simulink model "finaltuned"  (R2021a)
settings: Solver=FixedStepAuto  StartTime=0.0  StopTime=60  RelTol=1e-3  EnableMultiTasking=on
libraries: arduinolib x6
settings Model: SILPILModeSetting=veronly  ExtModeTrigDuration=2  Creator=admin  LastModifiedBy=admin
settings OptimizationCC: EnhancedBackFolding=on  PassReuseOutputArgsAs=Individual arguments  ZeroExternalMemoryAtStartup=off  ZeroInternalMemoryAtStartup=off  MaxStackSize=64  OptimizeBlockOrder=speed  DifferentSizesBufferReuse=on  OptimizationCustomize=off  EfficientTunableParamExpr=on
settings DebuggingCC: ParameterTunabilityLossMsg=error
settings HardwareCC: ProdBitPerPointer=32  ProdBitPerSizeT=32  ProdBitPerPtrDiffT=32  ProdLargestAtomicInteger=Long  ProdLargestAtomicFloat=Double  ProdWordSize=32  ProdHWDeviceType=ARM Compatible->ARM Cortex
settings SFSimCC: MATLABDynamicMemAlloc=off
settings RTWCC: SystemTargetFile=ert.tlc  HardwareBoard=Arduino Due  TemplateMakefile=ert_default_tmf  Toolchain=Arduino ARM  BuildConfiguration=Faster Runs
settings CodeAppCC: ForceParamTrailComments=on  IgnoreCustomStorageClasses=off  OperatorAnnotations=on  SimulinkDataObjDesc=on  SFDataObjDesc=on  InsertBlockDesc=on
settings ERTTargetCC: SupportContinuousTime=on  SupportVariableSizeSignals=on  ExtModeTransport=3  ExtModeStaticAlloc=on  ExtModeStaticAllocSize=24576  ExtModeMexFile=ext_xcp  ExtModeIntrfLevel=Level2 - Open

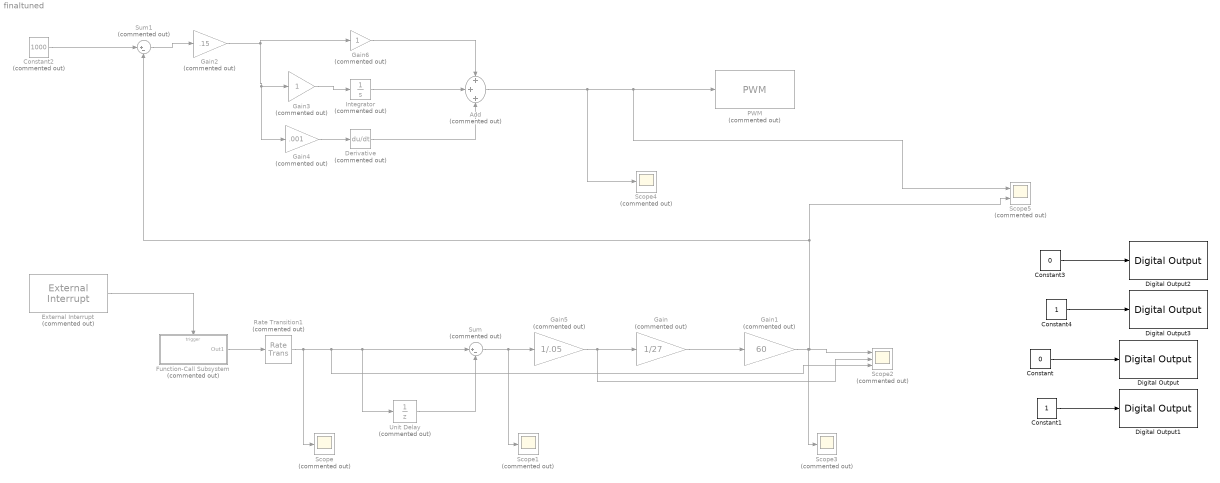
== system finaltuned ==
  Add : Sum  Commented=on  Inputs=+++
  Constant : Constant  Value=0
  Constant1 : Constant
  Constant2 : Constant  Commented=on  Value=1000  SampleTime=-1
  Constant3 : Constant  Value=0
  Constant4 : Constant
  Derivative : Derivative  Commented=on
  Digital Output : arduinolib/Digital Output  pinNumber=5  Direction=output  blockPlatform=arduino
  Digital Output1 : arduinolib/Digital Output  pinNumber=6  Direction=output  blockPlatform=arduino
  Digital Output2 : arduinolib/Digital Output  pinNumber=8  Direction=output  blockPlatform=arduino
  Digital Output3 : arduinolib/Digital Output  pinNumber=9  Direction=output  blockPlatform=arduino
  External Interrupt : arduinolib/External Interrupt  Commented=on  Pin=2  PullUp=off  Mode=RISING  InterruptSimulationInput=off
      settings: SourceProductBaseCode=ARDUINO
  Function-Call Subsystem : Subsystem  Commented=on  TreatAsAtomicUnit=on
  Gain : Gain  Commented=on  Gain=1/27
  Gain1 : Gain  Commented=on  Gain=60
  Gain2 : Gain  Commented=on  Gain=.15
  Gain3 : Gain  Commented=on
  Gain4 : Gain  Commented=on  Gain=.001
  Gain5 : Gain  Commented=on  Gain=1/.05
  Gain6 : Gain  Commented=on
  Integrator : Integrator  Commented=on
  PWM : arduinolib/PWM  Commented=on  pinNumber=4  frequencyType=Default  desiredFrequency=490.2  achievableFrequency=490.2
  Rate Transition1 : RateTransition  Commented=on  Deterministic=off
  Scope{,1,3..4} (4 alike) : Scope  Commented=on
  Scope2 : Scope  Commented=on  NumInputPorts=3
  Scope5 : Scope  Commented=on  NumInputPorts=2
  Sum : Sum  Commented=on  Inputs=|+-
  Sum1 : Sum  Commented=on  Inputs=|+-
  Unit Delay : UnitDelay  Commented=on  SampleTime=.05  HasFrameUpgradeWarning=on
  wires:
  Gain1/1 -> Scope3/1, Scope2/1, Scope5/2, Sum1/2
  Rate Transition1/1 -> Scope2/3, Unit Delay/1, Sum/1, Scope/1
  Unit Delay/1 -> Sum/2
  Sum/1 -> Scope1/1, Gain5/1
  Function-Call Subsystem/1(Out1) -> Rate Transition1/1
  External Interrupt/1 -> Function-Call Subsystem/Trigger
  Gain/1 -> Gain1/1
  Constant1/1 -> Digital Output1/1
  Constant/1 -> Digital Output/1
  Constant2/1 -> Sum1/1
  Sum1/1 -> Gain2/1
  Gain2/1 -> Gain4/1, Gain3/1, Gain6/1
  Gain3/1 -> Integrator/1
  Gain4/1 -> Derivative/1
  Integrator/1 -> Add/2
  Derivative/1 -> Add/3
  Add/1 -> Scope4/1, Scope5/1, PWM/1
  Gain5/1 -> Scope2/2, Gain/1
  Gain6/1 -> Add/1
  Constant3/1 -> Digital Output2/1
  Constant4/1 -> Digital Output3/1

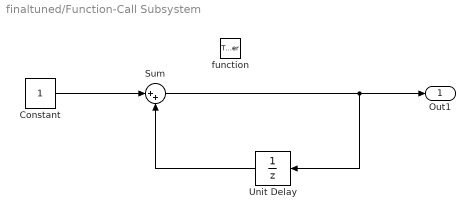
== system finaltuned/Function-Call Subsystem ==
  function : TriggerPort  TriggerType=function-call  VariantControl=(inherit)
  Constant : Constant  SampleTime=-1
  Sum : Sum  Inputs=|++
  Unit Delay : UnitDelay  SampleTime=-1  HasFrameUpgradeWarning=on
  Out1 : Outport  VectorParamsAs1DForOutWhenUnconnected=off
  wires:
  Unit Delay/1 -> Sum/2
  Constant/1 -> Sum/1
  Sum/1 -> Unit Delay/1, Out1/1
